simulink model "Test"  (R2024a)
settings: Solver=VariableStepAuto  StartTime=0.0  StopTime=2000  RelTol=1e-3
values from neighbouring files (symbols this model uses):
  a = exp(-plant.Ts/plant.tau)    [Main.m]
  g = b * 1.7    [Main.m]
undefined symbols (not defined in the file or in its folder): beta1, beta2, sigbuilder_block, TIME_DELAY
libraries: simulink x4, slpidlib x1, rllib x1
settings Model: Creator=rajeshs  LastModifiedBy=admin
settings SolverCC: AlgebraicLoopSolver=TrustRegion
settings DebuggingCC: UnconnectedInputMsg=warning  UnconnectedOutputMsg=warning  UnconnectedLineMsg=warning
settings ModelReferenceCC: EnableRefExpFcnMdlSchedulingChecks=on
settings SFSimCC: CustomCodeUndefinedFunction=UseInterfaceOnly
settings RTWCC: GPUComputeCapability=3.5

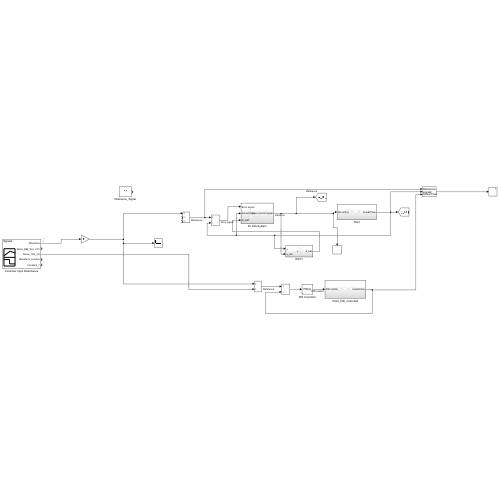
[thumbnail: Simulink's stored preview of the top-level diagram]
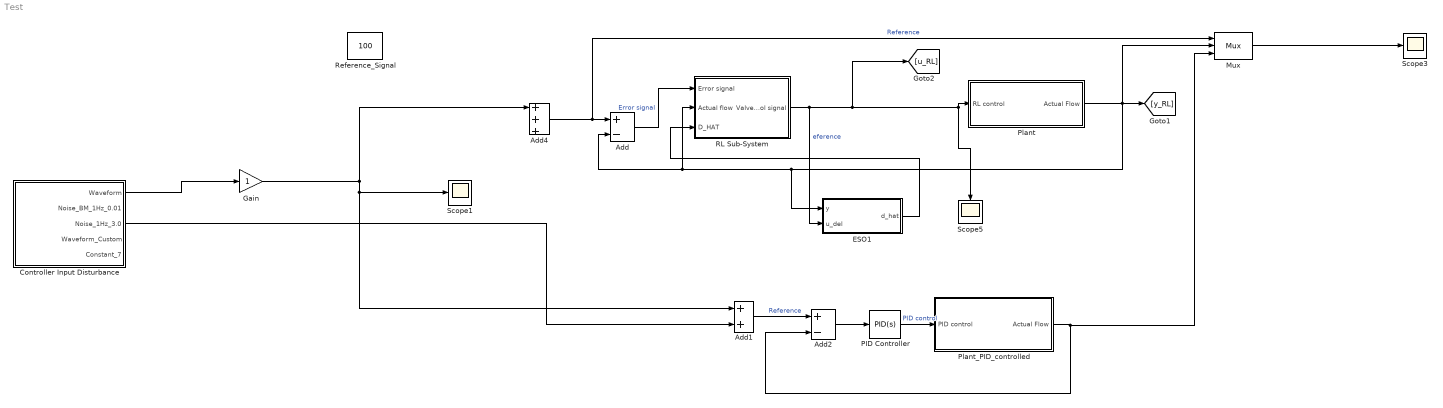
== system Test ==
  Add : Sum  Inputs=+-
  Add1 : Sum
  Add2 : Sum  Inputs=+-
  Add4 : Sum  Inputs=+++
  Controller Input Disturbance : Subsystem  Tag=STV Subsys  LoadFcn=sigbuilder_block('load');  StartFcn=sigbuilder_block('start');  StopFcn=sigbuilder_block('stop');  ClipboardFcn=sigbuilder_block('clipboard');  mask(Sigbuilder block){tuvar=[0:10]}
      mask help: Simulink:masks:SigbuilderBlock_MD
      mask init:
      | if ~strcmp(get_param(bdroot(gcbh),'SimulationStatus'),'stopped') tuvar = sigbuilder_block('maskInit'); end
      settings: CopyFcn=sigbuilder_block('copy');  DeleteFcn=sigbuilder_block('delete');  ModelCloseFcn=sigbuilder_block('modelClose');  PreSaveFcn=sigbuilder_block('preSave');  PauseFcn=sigbuilder_block('pause');  ContinueFcn=sigbuilder_block('continue');  NameChangeFcn=sigbuilder_block('namechange');  OpenFcn=sigbuilder_block('open',[0 0 1440 681 ]);  CloseFcn=sigbuilder_block('close');
      mask Display: plot(0, 0, 100, 100,[2, 2, 32, 32, 2], [68, 8, 8, 68, 68],[32, 2], [38, 38], [32, 19, 2],[53, 60, 44], [32, 17, 17, 2],[16, 16, 31, 31]);txt = getActiveGroup(gcbh);text(2, 100, txt,'verticalAlignment', 'top');
  ESO1 : Subsystem
  Gain : Gain
  Mux : Mux  Inputs=3
      settings: DisplayOption=signals
  PID Controller : slpidlib/PID Controller  Controller=PID  Form=Parallel  TimeDomain=Continuous-time  UseExternalTs=off  SampleTime=-1  IntegratorMethod=Forward Euler  FilterMethod=Forward Euler  ControllerParametersSource=internal  P=0.3631  I=0.0045  UseKiTs=off  D=-1.7202  UseExternalDerivativeSource=off  N=0.0114  UseFilter=on  TunerSelectOption=Transfer Function Based (PID Tuner App)  InitialConditionSource=internal  InitialConditionForIntegrator=0  InitialConditionForFilter=0  DifferentiatorICPrevScaledInput=0  ExternalReset=none  TrackingMode=off  Kt=1  LimitOutput=off  SatLimitsSource=internal  UpperSaturationLimit=inf  LowerSaturationLimit=-inf  LinearizeAsGain=on  AntiWindupMode=none  Kb=1  LimitIntegrator=off  UpperIntegratorSaturationLimit=inf  LowerIntegratorSaturationLimit=-inf  POutMin=[]  POutMax=[]  IOutMin=[]  IOutMax=[]  DOutMin=[]  DOutMax=[]  NOutMin=[]  NOutMax=[]  SumOutMin=[]  SumOutMax=[]  SaturationOutMin=[]  SaturationOutMax=[]  PParamMin=[]  PParamMax=[]  IParamMin=[]  IParamMax=[]  DParamMin=[]  DParamMax=[]  NParamMin=[]  NParamMax=[]  KbParamMin=[]  KbParamMax=[]  KtParamMin=[]  KtParamMax=[]  KbOutMin=[]  KbOutMax=[]  KtOutMin=[]  KtOutMax=[]  IntegratorOutMin=[]  IntegratorOutMax=[]  FilterOutMin=[]  FilterOutMax=[]  SumI1OutMin=[]  SumI1OutMax=[]  SumI2OutMin=[]  SumI2OutMax=[]  SumI3OutMin=[]  SumI3OutMax=[]  SumI4OutMin=[]  SumI4OutMax=[]  SumDOutMin=[]  SumDOutMax=[]  DifferentiatorOutMin=[]  DifferentiatorOutMax=[]  FilterDiffOutCoefMin=[]  FilterDiffOutCoefMax=[]  ReciprocalOutMin=[]  ReciprocalOutMax=[]  SumDenOutMin=[]  SumDenOutMax=[]  SumNumOutMin=[]  SumNumOutMax=[]  DivideOutMin=[]  DivideOutMax=[]  UdiffTsProdOutMin=[]  UdiffTsProdOutMax=[]  NTsProdOutMin=[]  NTsProdOutMax=[]  UintegralTsProdOutMin=[]  UintegralTsProdOutMax=[]  UngainTsProdOutMin=[]  UngainTsProdOutMax=[]  ClampingZeroOutDataTypeStr=Inherit: Inherit via back propagation  ClampingZeroOutMin=[]  ClampingZeroOutMax=[]  FilterDenConstantOutDataTypeStr=Inherit: Inherit via back propagation  FilterDenConstantOutMin=[]  FilterDenConstantOutMax=[]  PCopyOutDataTypeStr=Inherit: Inherit via back propagation  PCopyOutMin=[]  PCopyOutMax=[]  NCopyOutDataTypeStr=Inherit: Inherit via back propagation  NCopyOutMin=[]  NCopyOutMax=[]  IntegratorContinuousStateAttributes=''  IntegratorStateMustResolveToSignalObject=off  IntegratorRTWStateStorageClass=Auto  FilterContinuousStateAttributes=''  FilterStateMustResolveToSignalObject=off  FilterRTWStateStorageClass=Auto  ParallelPVariant=InternalParameters  IdealPVariant=Disabled  IVariant=InternalParameters  DVariant=InternalParameters  IntegratorVariant=Continuous  SatVariant=Disabled  AWVariant=Passthrough  PCopyVariant=Disabled  TRVariant=Disabled  FdbkBlocksVariant=Forward  IdealPFdbkVariant=Disabled  SatFdbkVariant=Disabled  DerivativeFilterVariant=ContFilter  NVariant=InternalParameters  NCopyVariant=Disabled  FilterICVariant=InternalICsFilter  IntegratorICVariant=InternalICs  ExternalResetVariant=Disabled  TRSumVariant=Passthrough  SumFdbkVariant=Disabled  SumVariant=Sum_PID  TsampFilterVariant=InternalTs  TsampNgainVariant=Passthrough  TsampIntegralVariant=Disabled_SignalSpec  ExternalSaturationOutDataTypeStr=Inherit: Same as second input  DerivativeSourceVariant=ErrorSignal
  Plant : Subsystem
  Plant_PID_controlled : Subsystem
  RL Sub-System : Subsystem
  Reference_Signal : Constant  Value=100
  Scope1 : Scope
  Scope3 : Scope
  Scope5 : Scope
  wires:
  Add/1 -> RL Sub-System/1(Error signal)  "Error signal"
  Mux/1 -> Scope3/1
  Add4/1 -> Mux/1, Add/1  "Reference"
  RL Sub-System/1(Valve control signal) -> ESO1/2(u_del), Plant/1(RL control), Scope5/1, [u_RL]  "eference"
  Plant/1(Actual Flow) -> ESO1/1(y), RL Sub-System/2(Actual flow), Add/2, Mux/2, [y_RL]
  Controller Input Disturbance/1(Waveform) -> Gain/1
  Plant_PID_controlled/1(Actual Flow) -> Mux/3, Add2/2
  PID Controller/1 -> Plant_PID_controlled/1(PID control)  "PID control"
  Add2/1 -> PID Controller/1
  Add1/1 -> Add2/1  "Reference"
  Gain/1 -> Add4/1, Scope1/1, Add1/1
  Controller Input Disturbance/3(Noise_1Hz_3.0) -> Add1/2
  ESO1/1(d_hat) -> RL Sub-System/3(D_HAT)

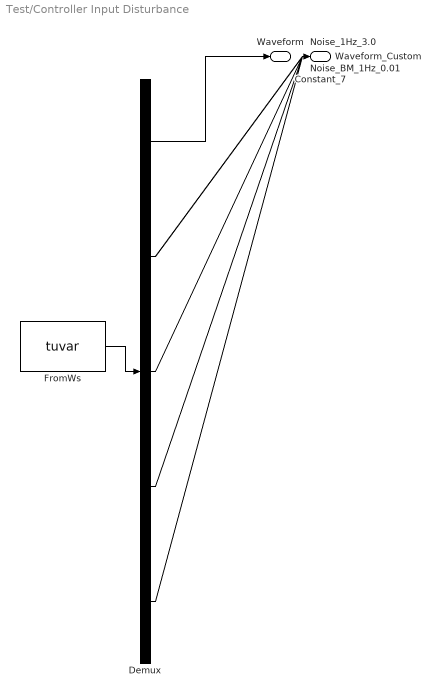
== system Test/Controller Input Disturbance ==
  Demux : Demux  Tag=STV Demux  Outputs=5
      settings: DisplayOption=none
  FromWs : FromWorkspace  Tag=STV FromWs  VariableName=tuvar
      SigBuilderData=|
      | common.afterFinalStr = 'Extrapolate'
      | common.sampleTime = 0
      | dataSet.timeRange = [0 2000]
      | dataSet.name = 'Signals'
      | sbobj.Groups.Name = 'Signals'
      | sbobj.Groups.Signals(1).Name = 'Waveform'
      | sbobj.Groups.Signals(1).XData = [0 752 752 1500 1500 1750 1750 2000]
      | sbobj.Groups.Signals(1).YData = [100 100 25 25 75 75 25 25]
      | sbobj.Groups.Signals(2).Name = 'Noise_BM_1Hz_0.01'
      | sbobj.Groups.Signals(2).XData = [0 1 2 3 4 5 6 7 8 9 10 11 ... (2001 elements, 1x2001)]
      | sbobj.Groups.Signals(2).YData = [0.0109017282673 -0.00358703225346 -0.0012992763049 0.00733737523776 0.00120331570317 0.0113633128469 -0.00686773118719 0.00471682863443 0.00288342465456 0.0139185483505 -0.0134550201016 7.47406191734e-06 ... (2001 elements, 1x2001)]
      | sbobj.Groups.Signals(3).Name = 'Noise_1Hz_3.0'
      | sbobj.Groups.Signals(3).XData = [0 1 2 3 4 5 6 7 8 9 10 11 ... (2001 elements, 1x2001)]
      | sbobj.Groups.Signals(3).YData = [-1.22103016093 -2.32126408989 6.42034479721 -4.13028289214 0.366124868815 1.68201285192 -3.06458126709 -0.0302582378605 -4.3152453304 1.33545254952 0.451492702689 0.846422939597 ... (2001 elements, 1x2001)]
      | sbobj.Groups.Signals(4).Name = 'Waveform_Custom'
      | sbobj.Groups.Signals(4).XData = [0 100 110 200 290 398 500 600 1000 1050 1225 1400 1500 2000]
      | sbobj.Groups.Signals(4).YData = [75 75 100 100 100 20 20 75 75 10 10 100 100 5]
      | sbobj.Groups.Signals(5).Name = 'Constant_7'
      | sbobj.Groups.Signals(5).XData = [0 2000]
      | sbobj.Groups.Signals(5).YData = [100 100]
      | sbobj.Groups.TimeRange = [0 2000]
  Waveform : Outport  Tag=STV Outport  VectorParamsAs1DForOutWhenUnconnected=off
  Noise_BM_1Hz_0.01 : Outport  Tag=STV Outport  Port=2  VectorParamsAs1DForOutWhenUnconnected=off
  Noise_1Hz_3.0 : Outport  Tag=STV Outport  Port=3  VectorParamsAs1DForOutWhenUnconnected=off
  Waveform_Custom : Outport  Tag=STV Outport  Port=4  VectorParamsAs1DForOutWhenUnconnected=off
  Constant_7 : Outport  Tag=STV Outport  Port=5  VectorParamsAs1DForOutWhenUnconnected=off
  wires:
  Demux/1 -> Waveform/1
  FromWs/1 -> Demux/1
  Demux/2 -> Noise_BM_1Hz_0.01/1
  Demux/3 -> Noise_1Hz_3.0/1
  Demux/4 -> Waveform_Custom/1
  Demux/5 -> Constant_7/1

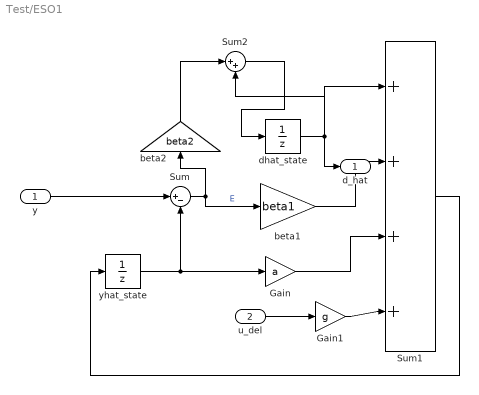
== system Test/ESO1 ==
  y : Inport
  u_del : Inport  Port=2
  Gain : Gain  Gain=a
  Gain1 : Gain  Gain=g
  Sum : Sum  Inputs=|+-
  Sum1 : Sum  Inputs=|++++
  Sum2 : Sum  Inputs=|++
  beta1 : Gain  Gain=beta1
  beta2 : Gain  Gain=beta2
  dhat_state : UnitDelay  SampleTime=-1  HasFrameUpgradeWarning=on
  yhat_state : UnitDelay  SampleTime=-1  HasFrameUpgradeWarning=on
  d_hat : Outport
  wires:
  yhat_state/1 -> Gain/1, Sum/2
  y/1 -> Sum/1
  Sum/1 -> beta2/1, beta1/1  "E"
  u_del/1 -> Gain1/1
  Sum1/1 -> yhat_state/1
  Gain1/1 -> Sum1/4
  Gain/1 -> Sum1/3
  beta1/1 -> Sum1/2
  dhat_state/1 -> d_hat/1, Sum1/1, Sum2/2
  beta2/1 -> Sum2/1
  Sum2/1 -> dhat_state/1

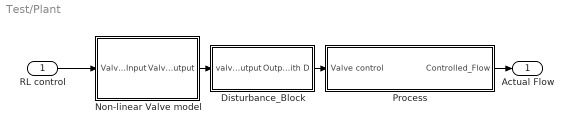
== system Test/Plant ==
  RL control : Inport
  Disturbance_Block : Subsystem
  Non-linear Valve model : Subsystem
  Process : Subsystem
  Actual Flow : Outport  VectorParamsAs1DForOutWhenUnconnected=off
  wires:
  RL control/1 -> Non-linear Valve model/1(ValveInput)
  Process/1(Controlled_Flow) -> Actual Flow/1
  Non-linear Valve model/1(ValveOutput) -> Disturbance_Block/1(valve Output)
  Disturbance_Block/1(Output with D) -> Process/1(Valve control)

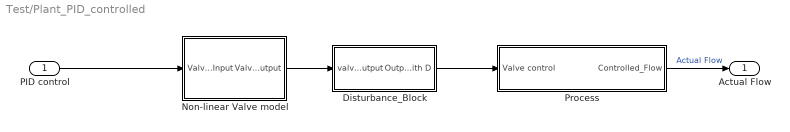
== system Test/Plant_PID_controlled ==
  PID control : Inport
  Disturbance_Block : Subsystem
  Non-linear Valve model : Subsystem
  Process : Subsystem
  Actual Flow : Outport  VectorParamsAs1DForOutWhenUnconnected=off
  wires:
  Process/1(Controlled_Flow) -> Actual Flow/1  "Actual Flow"
  PID control/1 -> Non-linear Valve model/1(ValveInput)
  Non-linear Valve model/1(ValveOutput) -> Disturbance_Block/1(valve Output)
  Disturbance_Block/1(Output with D) -> Process/1(Valve control)

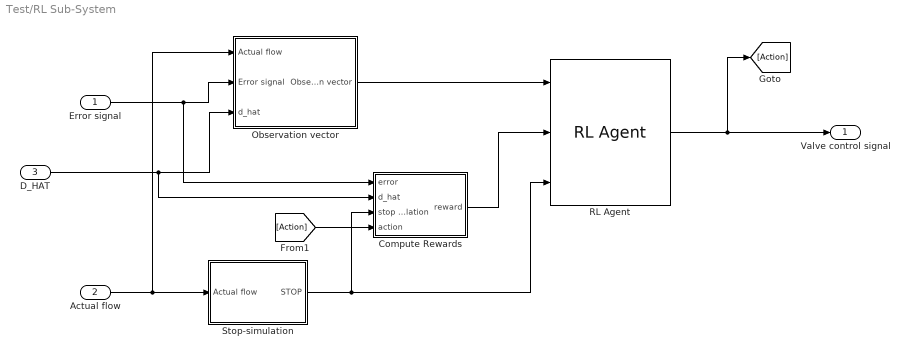
== system Test/RL Sub-System ==
  Error signal : Inport
  Actual flow : Inport  Port=2
  D_HAT : Inport  Port=3
  Compute Rewards : Subsystem
  Observation vector : Subsystem
  RL Agent : rllib/RL Agent  Agent=agent  ExternalActionAsInput=off  ProvideLastAction=off  ProvideCumRwd=off  TreatAsDirectFeedthrough=on  UseStrictObservationDataTypes=off
  Stop-simulation : Subsystem
  Valve control signal : Outport  VectorParamsAs1DForOutWhenUnconnected=off
  wires:
  Stop-simulation/1(STOP) -> RL Agent/3, Compute Rewards/3(stop simulation)
  Error signal/1 -> Observation vector/2(Error signal), Compute Rewards/1(error)
  Observation vector/1(Observation vector) -> RL Agent/1
  RL Agent/1 -> [Action], Valve control signal/1
  Actual flow/1 -> Observation vector/1(Actual flow), Stop-simulation/1(Actual flow)
  Compute Rewards/1(reward) -> RL Agent/2
  [Action] -> Compute Rewards/4(action)
  D_HAT/1 -> Compute Rewards/2(d_hat), Observation vector/3(d_hat)

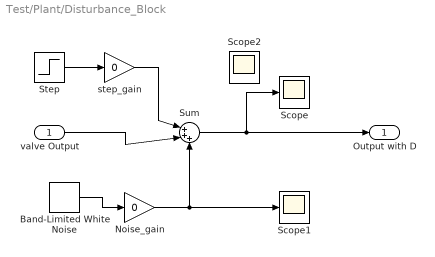
== system Test/Plant/Disturbance_Block ==
  valve Output : Inport
  Band-Limited White Noise : simulink/Sources/Band-Limited White Noise  Cov=[0.1]  Ts=1  seed=[23341]
  Noise_gain : Gain  Gain=0
  Scope : Scope
  Scope1 : Scope
  Scope2 : Scope
  Step : Step  Time=800  SampleTime=0
  Sum : Sum  Inputs=|+++
  step_gain : Gain  Gain=0
  Output with D : Outport
  wires:
  Step/1 -> step_gain/1
  valve Output/1 -> Sum/2
  Band-Limited White Noise/1 -> Noise_gain/1
  Sum/1 -> Scope/1, Output with D/1
  Noise_gain/1 -> Scope1/1, Sum/3
  step_gain/1 -> Sum/1

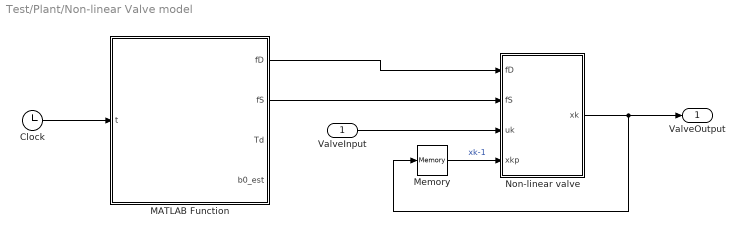
== system Test/Plant/Non-linear Valve model ==
  ValveInput : Inport
  Clock : Clock
  MATLAB Function : MATLAB Function  TreatAsAtomicUnit=on
  Memory : Memory
  Non-linear valve : MATLAB Function  TreatAsAtomicUnit=on
  ValveOutput : Outport  VectorParamsAs1DForOutWhenUnconnected=off
  wires:
  Non-linear valve/1(xk) -> ValveOutput/1, Memory/1
  Memory/1 -> Non-linear valve/4(xkp)  "xk-1"
  ValveInput/1 -> Non-linear valve/3(uk)
  Clock/1 -> MATLAB Function/1(t)
  MATLAB Function/2(fS) -> Non-linear valve/2(fS)
  MATLAB Function/1(fD) -> Non-linear valve/1(fD)

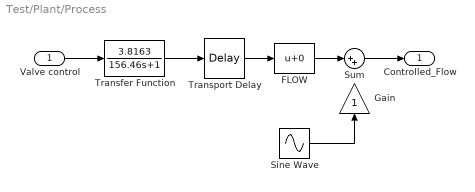
== system Test/Plant/Process ==
  Valve control : Inport
  FLOW : Bias  SaturateOnIntegerOverflow=off
  Gain : Gain
  Sine Wave : Sin  Amplitude=0.9  Frequency=0.1  SampleTime=0
  Sum : Sum  Inputs=|++
  Transfer Function : TransferFcn  Numerator=[3.8163]  Denominator=[156.46 1]
  "Transport Delay " : TransportDelay  DelayTime=TIME_DELAY
  Controlled_Flow : Outport  VectorParamsAs1DForOutWhenUnconnected=off
  wires:
  "Transport Delay "/1 -> FLOW/1
  Sum/1 -> Controlled_Flow/1
  FLOW/1 -> Sum/1
  Transfer Function/1 -> "Transport Delay "/1
  Valve control/1 -> Transfer Function/1
  Sine Wave/1 -> Gain/1

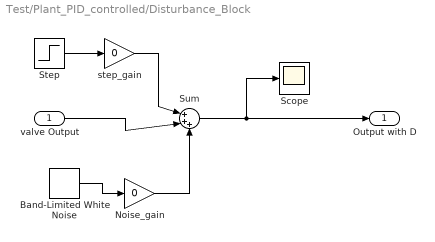
== system Test/Plant_PID_controlled/Disturbance_Block ==
  valve Output : Inport
  Band-Limited White Noise : simulink/Sources/Band-Limited White Noise  Cov=[0.1]  Ts=1  seed=[23341]
  Noise_gain : Gain  Gain=0
  Scope : Scope
  Step : Step  Time=800  SampleTime=0
  Sum : Sum  Inputs=|+++
  step_gain : Gain  Gain=0
  Output with D : Outport
  wires:
  Step/1 -> step_gain/1
  step_gain/1 -> Sum/1
  valve Output/1 -> Sum/2
  Band-Limited White Noise/1 -> Noise_gain/1
  Sum/1 -> Scope/1, Output with D/1
  Noise_gain/1 -> Sum/3

== system Test/Plant_PID_controlled/Non-linear Valve model ==
  ValveInput : Inport
  Memory : Memory
  Non-linear valve : MATLAB Function  TreatAsAtomicUnit=on
  ValveOutput : Outport  VectorParamsAs1DForOutWhenUnconnected=off
  wires:
  Non-linear valve/1(xk) -> ValveOutput/1, Memory/1
  Memory/1 -> Non-linear valve/2(xkp)  "xk-1"
  ValveInput/1 -> Non-linear valve/1(uk)

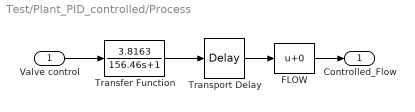
== system Test/Plant_PID_controlled/Process ==
  Valve control : Inport
  FLOW : Bias  SaturateOnIntegerOverflow=off
  Transfer Function : TransferFcn  Numerator=[3.8163]  Denominator=[156.46 1]
  "Transport Delay " : TransportDelay  DelayTime=TIME_DELAY
  Controlled_Flow : Outport  VectorParamsAs1DForOutWhenUnconnected=off
  wires:
  FLOW/1 -> Controlled_Flow/1
  Transfer Function/1 -> "Transport Delay "/1
  Valve control/1 -> Transfer Function/1
  "Transport Delay "/1 -> FLOW/1

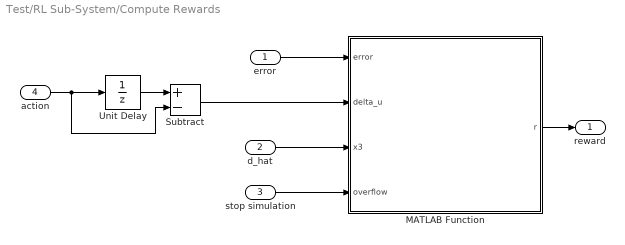
== system Test/RL Sub-System/Compute Rewards ==
  error : Inport
  d_hat : Inport  Port=2
  stop simulation : Inport  Port=3
  action : Inport  Port=4
  MATLAB Function : MATLAB Function  TreatAsAtomicUnit=on
  Subtract : Sum  Inputs=+-
  Unit Delay : UnitDelay  SampleTime=-1  HasFrameUpgradeWarning=on
  reward : Outport
  wires:
  error/1 -> MATLAB Function/1(error)
  d_hat/1 -> MATLAB Function/3(x3)
  stop simulation/1 -> MATLAB Function/4(overflow)
  action/1 -> Subtract/2, Unit Delay/1
  Unit Delay/1 -> Subtract/1
  Subtract/1 -> MATLAB Function/2(delta_u)
  MATLAB Function/1(r) -> reward/1

== system Test/RL Sub-System/Observation vector ==
  Actual flow : Inport
  Error signal : Inport  Port=2
  d_hat : Inport  Port=3
  Mux1 : Mux  Inputs=3
  Observation vector : Outport  VectorParamsAs1DForOutWhenUnconnected=off
  wires:
  Error signal/1 -> Mux1/2
  Mux1/1 -> Observation vector/1
  Actual flow/1 -> Mux1/1
  d_hat/1 -> Mux1/3

== system Test/RL Sub-System/Stop-simulation ==
  Actual flow : Inport
  Compare To Constant : simulink/Logic and Bit Operations/Compare To Constant  relop=>  const=200  OutDataTypeStr=boolean
  Compare To Constant2 : simulink/Logic and Bit Operations/Compare To Constant  relop=<  const=0  OutDataTypeStr=boolean
  OR : Logic  Operator=OR  IconShape=distinctive  AllPortsSameDT=off  OutDataTypeStr=boolean
  STOP : Outport  VectorParamsAs1DForOutWhenUnconnected=off
  wires:
  Compare To Constant/1 -> OR/1
  Actual flow/1 -> Compare To Constant/1, Compare To Constant2/1
  Compare To Constant2/1 -> OR/2
  OR/1 -> STOP/1

== matlab function Test/RL Sub-System/Compute Rewards/MATLAB Function ==
  data: error input; r output; delta_u input; x3 input; overflow input
function r = compute_reward(error, delta_u, x3, overflow)

% وزن‌دهی‌ها
w1 = 2.2;      % برای خطا
w2 = 0.2;    % برای تغییرات کنترل
w3 = 0.3;    % برای تخمین اغتشاش x3
w4 = 100;    % برای overflow

% محدودسازی x3 به بازه [-5, 5] (برای ثبات عددی)
x3 = max(min(x3, 5), -5);

% محاسبه پاداش
r = - w1 * abs(error) ...
    - w2 * abs(delta_u) ...
    - w3 * abs(x3);

% اعمال جریمه overflow
if overflow
    r = r - w4;
end

if abs(error) < 0.5 && abs(delta_u) < 0.1
    r = r + 5;  % تشویق رفتار خیلی خوب
end

== matlab function Test/Plant/Non-linear Valve model/Non-linear valve ==
  data: fD input; fS input; uk input; xk output; xkp input
function xk = fcn(fD, fS, uk, xkp)
% -------------------------------------------------------------------------

% -------------------------------------------------------------------------
% uk - fD   if uk - xk−1 > fS
% uk + fD   if uk - xk−1 < -fS
% xk - 1    if |uk - xk−1| < fS
% -------------------------------------------------------------------------
% Graded Learning Stages:
% GRADE_I    TIME_DELAY=0.1; fS = 8.4/10; fD = 3.5243/10 
% GRADE_II   TIME_DELAY=0.5; fS = 8.4/5; fD = 3.5243/5
% GRADE_III  TIME_DELAY=1.5; fS = 8.4/2; fD = 3.5243/2
% GRADE_IV   TIME_DELAY=1.5; fS = 8.4/1.5; fD = 3.5243/1.5
% GRADE_IV   TIME_DELAY=1.5, fS/1.5 and fD/1.5
% GRADE_V    TIME_DELAY=2.0, fS/1.5 and fD/1.5
% GRADE_VI   TIME_DELAY=2.5, fS/1.0 and fD/1.0
% -------------------------------------------------------------------------

    % uk = uk(1,1)/1.7;
     
    t_xk = 0.0;
   
    if ((1.7*uk-xkp) > fS)
        t_xk = 1.7*uk - fD;
    elseif ((1.7*uk-xkp) < -1*fS)
        t_xk = 1.7*uk + fD;
    elseif (abs(1.7*uk-xkp) < fS)
        t_xk = xkp;
    end
    
xk = t_xk;

== matlab function Test/Plant/Non-linear Valve model/MATLAB Function ==
  data: fD output; t input; fS output; Td output; b0_est output
function [fD, fS, Td, b0_est] = param_scheduler(t) %#codegen
% t: simulation time from Clock
% Outputs:
%  fS, fD : stiction/friction thresholds (valve)
%  Td     : time delay (for a Transport/Variable Delay block)
%  b0_est : nominal plant/actuator gain used by ADRC (optional)

% --- Base values (Grade I) ---
fs1 = 8.4/1;     fd1 = 3.5243/1;   Td1 = 0.5;   b01 = 1.0;

% --- Jump 1 (stronger friction + larger delay) ---
fs2 = 4*fs1;      fd2 = 4*fd1;       Td2 = 2.0;   b02 = 0.8*b01;

% --- Jump 2 (different regime) ---
fs3 = 1.5*fs1;    fd3 = 1.5*fd1;     Td3 = 1.0;   b03 = 1.2*b01;

% --- Defaults (must assign for codegen) ---
fS = fs1; fD = fd1; Td = Td1; b0_est = b01;

% --- Schedule by time (edit breakpoints as you like) ---
% if t >= 400 && t < 600
%     fS = fs2; fD = fd2; Td = Td2; b0_est = b02;
% elseif t >= 1600
%     fS = fs3; fD = fd3; Td = Td3; b0_est = b03;
% end
end

== matlab function Test/Plant_PID_controlled/Non-linear Valve model/Non-linear valve ==
  data: uk input; xk output; xkp input
function xk = fcn(uk, xkp)
% ----------------------------------------------------------------------------------------
% PID EVALUATION circuit Plant Model (RLVC2 | Verified 15-Jul-2020)
% Non-Linear valve model: Capaci and Scali (2018)
% Friction values conform to benchmark flow rates used in Capaci (2016)
% ----------------------------------------------------------------------------------------
% uk - fD   if uk - xk−1 > fS
% uk + fD   if uk - xk−1 < -fS
% xk - 1    if |uk - xk−1| < fS
% ----------------------------------------------------------------------------------------

    fS = 8.4;
    fD = 3.5243;
        
    t_xk = 0.0;
   
    if ((uk-xkp) > fS)
        t_xk = uk - fD;
    elseif ((uk-xkp) < -1*fS)
        t_xk = uk + fD;
    elseif (abs(uk-xkp) < fS)
        t_xk = xkp;
    end
    
xk = t_xk;
